simulink model "EKF_SIL_02"  (R2015a)
settings: Solver=ode45  StartTime=0.0  StopTime=totalSimulationTime  RelTol=1e-3
model workspace: external: MATLAB File Init_Model_02_Simulink.m (data not in the file)
undefined symbols (not defined in the file): Cov_nu, Cov_r, e_force_x, e_force_y, e_force_z, ieps, ita, lenLinks, n, P_d, P_k, p_x, p_y, p_z, parameter_gravitation, rho, rho_c, sig_f, sig_tau, t_delta, t_Kalman, tau_1, tau_2, tau_3, U_n_d, W_0, X_a_0, x_d, x_k
libraries: simulink x9, aerolibtransform2 x3, dspmtrx3 x2, visionstatistics x1, aerolibutil x1, visionsinks x1
(part 5 of 5)

== matlab function EKF_SIL_02/EKF/Measurement Update/Create X from X_a/Create del_q [Intermediate stage]/MATLAB Function ==
  data: q input; CrossTensor output; flag input
%Inputs: q: quaternion vector
%        flag:0-cross;1-star
function CrossTensor  = fn_CrossTensor(q,flag)
    %#codegen
    CrossTensor = zeros(4,4);
    q_v = q(1:3);
    q_0 = q(4);    
    cross_q_v = fn_VectorToSkewSymmetricTensor(q_v);
    switch (flag)
        case 0
            CrossTensor = [-cross_q_v + q_0*eye(3,3), q_v;-q_v',q_0];
        case 1
            CrossTensor = [cross_q_v + q_0*eye(3,3), q_v;-q_v',q_0];
        otherwise
            
    end
end

== matlab function EKF_SIL_02/EKF/Predictor/Create State error covariance (P)/State Propagation/MATLAB Function ==
  data: X_a input; Phi output; n input; t_Kalman input; p input; M input
%Function: fn_Create_Phi()
%Inputs: X_a - 23-state vector,
%        n - angular velocity of spacecrafts,
%        t_delta - sampling time
%Outputs: [Phi] (State-propagation Matrix)
%Functionality: Generates the State Propagation matrix
%Author: Hrishik Mishra
function Phi  = fn_Create_Phi(X_a,n,t_Kalman,p,M)
    Phi_t = fn_Create_Phi_t(n,t_Kalman);
    Phi_r = fn_Create_Phi_r(X_a,p, t_Kalman);
    Phi = [Phi_r, zeros(6,6);zeros(6,6),Phi_t];

end
%Create state propagation matrix of the whole system

%Function: fn_Create_Phi_r()
%Inputs: X_a - 23-state vector,
%Outputs: [Phi_r] (State-propagation Matrix for Rotation component)
%Functionality: Generates the State Propagation matrix for Rotation
%component
%Author: Hrishik Mishra
function [Phi_r] = fn_Create_Phi_r(X_a,p,t_Kalman) 
    Phi_r = zeros(6,6);
    omega = X_a(5:7);
    M = fn_Create_M(p,omega);   
    
    A = [-fn_VectorToSkewSymmetricTensor(omega),0.5*eye(3,3);zeros(3,3),M];
    Phi_r = expm(A*t_Kalman);
%     phi_r11 = fn_Create_phi_r11(omega,t_delta);
%     phi_r12 = fn_Create_phi_r12(omega,M,t_delta);
%     phi_r22 = fn_Create_phi_r22(omega,t_delta,M);
%     phi_r13 = fn_Create_phi_r13(omega,t_delta,M,N);
%     phi_r23 = fn_Create_phi_r23(omega,t_delta,M,N);
%     Phi_r = [phi_r11, phi_r12, phi_r13;zeros(3,3),phi_r22,phi_r23;zeros(3,3),zeros(3,3),eye(3,3)];
%     

end
%Function: fn_Create_M()
%Inputs: p - Inertial ratios 
%        omega - angular velocity between Chaser Grasping frame and Chaser
%        CoM
%Outputs: M (Linearized model matrix for inertial parameters)
%Functionality: Generates M
%Author: Hrishik Mishra
function M = fn_Create_M(p,omega)
    %#Codegen
    
    M = [0, p(1)*omega(3), p(1)*omega(2); p(2)*omega(3), 0, p(2)*omega(1); p(3)*omega(2),p(3)*omega(1),0];
end
%Function: fn_Create_N()
%Inputs: omega - angular velocity between Chaser Grasping frame and Chaser
%        CoM
%Outputs: N (Linearized model matrix for inertial parameters)
%Functionality: Generates M
%Author: Hrishik Mishra
function N = fn_Create_N(omega)
%
    N = [omega(2)*omega(3), 0, 0; 0, omega(1)*omega(3), 0; 0, 0, omega(1)*omega(2)];
end

%%
%Function: fn_Create_Phi_t()
%Inputs: n - angular velocity of Chaser/Target (almost same)
%        t_delta - sampling time
%Outputs: Phi_t (State Transition Matrix for Translation component)
%Functionality: Generates Phi_t
%Author: Hrishik Mishra
function Phi_t = fn_Create_Phi_t(n,t_delta)
%
    Phi_t12 = [t_delta, n*t_delta^2,0;0, t_delta, 0;0,0,t_delta];
    Phi_t22 = eye(3,3) - 2*fn_VectorToSkewSymmetricTensor([0;0;n])*t_delta;
    
    Phi_t = [eye(3,3),Phi_t12;zeros(3,3),Phi_t22];
    
end

== matlab function EKF_SIL_02/EKF/Predictor/Create State error covariance (P)/Process noise covariance [rotational]/Process Noise covariance ==
  data: Phi input; Q_r output; unused1 input; t_delta input; tau input; unused input; p input
%Function: fn_Create_Q_r()
%Inputs: Phi - State Propagation Matrix for Rotational component
%        X - 23-state vector
%        t_delta - sampling time
%        tau - Torque disturbance
%        sig_p - Uncertainty in Inertial ratios (p)
%Outputs: Q_r (Rotation component Process noise)
%Functionality: Generates Q_r
%Author: Hrishik Mishra
function Q_r = fn_Create_Q_r(Phi,~, t_delta, tau,~,p)
    %#codegen
    J = fn_Create_J(p);
    Q_r11 = 0.25*fn_Create_Q_r11(Phi(1:3,4:6), J, t_delta, tau);
    Q_r12 = 0.5*fn_Create_Q_r12(Phi(1:3,4:6),Phi(4:6,4:6),J,t_delta,tau);
    Q_r22 = fn_Create_Q_r22(Phi(4:6,4:6),J,t_delta,tau);
    Q_r = [Q_r11, Q_r12;Q_r12' Q_r22];
    
end
%check if it is actually phi_r12 or phi_r11
function Q_r11 = fn_Create_Q_r11(phi_r12, J, t_delta, tau)
    Q_r11 = tau*phi_r12*J^2*phi_r12'*t_delta; 
end

function Q_r12 = fn_Create_Q_r12(phi_r12,phi_r22,J, t_delta, tau)
    Q_r12 = tau*phi_r12*J^2*phi_r22*t_delta;
end
function Q_r22 = fn_Create_Q_r22(phi_r22, J, t_delta, tau)
    Q_r22 = tau*phi_r22*J^2*phi_r22*t_delta;
end
%Function: fn_Create_J()
%Inputs: p: Inertial ratios
%Outputs: J (Inertial Ratio Matrix for omega_dot)
%Functionality: Generates J
%Author: Hrishik Mishra
function J = fn_Create_J(p)
    J = [1 0 0;0 (1-p(2))/(1+p(1)) 0;0 0 (1+p(3))/(1-p(1))];
end

== matlab function EKF_SIL_02/EKF/Predictor/Create State error covariance (P)/Process noise covariance [translational]/Process noise covariance [translational] ==
  data: t_Kalman input; Q_t_k output; n input; sigma_f input
%Function: fn_Create_Q_t_k()
%Inputs: t_delta: sampling time
%        sigma_f: variance of force perturbations
%Outputs: Q_t_k (Translational component Process noise)
%Functionality: Generates Q_t_k
%Author: Hrishik Mishra
function Q_t_k  = fn_Create_Q_t_k(t_Kalman, n,sigma_f)
    %#codegen

    Q_t11_k = [(t_Kalman^3)/3 + (2/5)*n^2*t_Kalman^5, (1/4)*(n - n^2)*t_Kalman^4, 0;(1/4)*(n - n^2)*t_Kalman^4, (t_Kalman^3)/3 - (4/15)*n^2*t_Kalman^5 0;0, 0, (t_Kalman^3)/3 - (1/15)*n^2*t_Kalman^5];
    Q_t12_k = [(t_Kalman^2)/2 + (1/3)*(n^2)*(t_Kalman^4), -(1/3)*n*(t_Kalman^3),0;(2/3)*(n - n^2)*t_Kalman^3, (1/2)*(t_Kalman^2) - (2/3)*(n^2)*(t_Kalman^4) 0;0 0 (1/2)*(t_Kalman^2) - (1/6)*(n^2)*(t_Kalman^4)];
    Q_t22_k = [t_Kalman + (n^2)*(t_Kalman^3), 0, 0;0, t_Kalman, 0;0, 0, t_Kalman - (1/3)*(n^2)*(t_Kalman^3)];

    Q_t_k = [Q_t11_k, Q_t12_k;Q_t12_k',Q_t22_k];

    Q_t_k = sigma_f*Q_t_k;
end

== matlab function EKF_SIL_02/EKF/Measurement Update/Update with K(k) and predict current state/Create observation/MATLAB Function ==
  data: q input; CrossTensor output; flag input
%Inputs: q: quaternion vector
%        flag:0-cross;1-star
function CrossTensor  = fn_CrossTensor(q,flag)
    %#codegen
    CrossTensor = zeros(4,4);
    q_v = q(1:3);
    q_0 = q(4);    
    cross_q_v = fn_VectorToSkewSymmetricTensor(q_v);
    switch (flag)
        case 0
            CrossTensor = [-cross_q_v + q_0*eye(3,3), q_v;-q_v',q_0];
        case 1
            CrossTensor = [cross_q_v + q_0*eye(3,3), q_v;-q_v',q_0];
        otherwise
            
    end
end

== matlab function EKF_SIL_02/EKF/Measurement Update/Update with K(k) and predict current state/Measurement noise covariance ==
  data: q_nominal input; S output; ita_nominal input; cov_r input; cov_nu input
%Function: fn_Create_S()
%Inputs: q_nominal: Quaternion between Chaser CoM and Target CoM
%        ita_nominal: Quaternion between Target CoM and Target grasping
%        frame
%        cov_r: position covariance due to camera
%        cov_nu: orientation covariance due to camera
%Outputs: S (Measurement noise covariance Matrix)
%Functionality: Generates S
%Author: Hrishik Mishra
function S   = fn_Create_S(q_nominal,ita_nominal,cov_r,cov_nu)
    %#codegen
    q_star = [-q_nominal(1:3);q_nominal(4)];
    ita_star = [-ita_nominal(1:3);ita_nominal(4)];
    Ita_Tensor = fn_CrossTensor(ita_star,0);
    Q_Tensor = fn_CrossTensor(q_star,1);
    T = [eye(3,3),zeros(3,1)]*Ita_Tensor*Q_Tensor;
    S = [cov_r,zeros(3,3);zeros(3,3), T*cov_nu*T'];
end

== matlab function EKF_SIL_02/EKF/Measurement Update/Update with K(k) and predict current state/Create observation/MATLAB Function2 ==
  data: q input; CrossTensor output; flag input
%Inputs: q: quaternion vector
%        flag:0-cross;1-star
function CrossTensor  = fn_CrossTensor(q,flag)
    %#codegen
    CrossTensor = zeros(4,4);
    q_v = q(1:3);
    q_0 = q(4);    
    cross_q_v = fn_VectorToSkewSymmetricTensor(q_v);
    switch (flag)
        case 0
            CrossTensor = [-cross_q_v + q_0*eye(3,3), q_v;-q_v',q_0];
        case 1
            CrossTensor = [cross_q_v + q_0*eye(3,3), q_v;-q_v',q_0];
        otherwise
            
    end
end

== matlab function EKF_SIL_02/EKF/Measurement Update/Update with K(k) and predict current state/Create h/Subsystem/MATLAB Function2 ==
  data: q input; CrossTensor output; flag input
%Inputs: q: quaternion vector
%        flag:0-cross;1-star
function CrossTensor  = fn_CrossTensor(q,flag)
    %#codegen
    CrossTensor = zeros(4,4);
    q_v = q(1:3);
    q_0 = q(4);    
    cross_q_v = fn_VectorToSkewSymmetricTensor(q_v);
    switch (flag)
        case 0
            CrossTensor = [-cross_q_v + q_0*eye(3,3), q_v;-q_v',q_0];
        case 1
            CrossTensor = [cross_q_v + q_0*eye(3,3), q_v;-q_v',q_0];
        otherwise
            
    end
end

== matlab function EKF_SIL_02/EKF/Measurement Update/Update with K(k) and predict current state/Create X_a from X/Create q_nominal /MATLAB Function2 ==
  data: q input; CrossTensor output; flag input
%Inputs: q: quaternion vector
%        flag:0-cross;1-star
function CrossTensor  = fn_CrossTensor(q,flag)
    %#codegen
    CrossTensor = zeros(4,4);
    q_v = q(1:3);
    q_0 = q(4);    
    cross_q_v = fn_VectorToSkewSymmetricTensor(q_v);
    switch (flag)
        case 0
            CrossTensor = [-cross_q_v + q_0*eye(3,3), q_v;-q_v',q_0];
        case 1
            CrossTensor = [cross_q_v + q_0*eye(3,3), q_v;-q_v',q_0];
        otherwise
            
    end
end

== matlab function EKF_SIL_02/EKF/OOSM_KF/OOSM_KF/Initialize OOSM/Create State error covariance (P)/Process noise covariance [rotational]/Process Noise covariance ==
  data: Phi input; Q_r output; unused1 input; t_delta input; tau input; unused input; p input
%Function: fn_Create_Q_r()
%Inputs: Phi - State Propagation Matrix for Rotational component
%        X - 23-state vector
%        t_delta - sampling time
%        tau - Torque disturbance
%        sig_p - Uncertainty in Inertial ratios (p)
%Outputs: Q_r (Rotation component Process noise)
%Functionality: Generates Q_r
%Author: Hrishik Mishra
function Q_r = fn_Create_Q_r(Phi,~, t_delta, tau,~,p)
    %#codegen
    J = fn_Create_J(p);
    Q_r11 = 0.25*fn_Create_Q_r11(Phi(1:3,4:6), J, t_delta, tau);
    Q_r12 = 0.5*fn_Create_Q_r12(Phi(1:3,4:6),Phi(4:6,4:6),J,t_delta,tau);
    Q_r22 = fn_Create_Q_r22(Phi(4:6,4:6),J,t_delta,tau);
    Q_r = [Q_r11, Q_r12;Q_r12' Q_r22];
    
end
%check if it is actually phi_r12 or phi_r11
function Q_r11 = fn_Create_Q_r11(phi_r12, J, t_delta, tau)
    Q_r11 = tau*phi_r12*J^2*phi_r12'*t_delta; 
end

function Q_r12 = fn_Create_Q_r12(phi_r12,phi_r22,J, t_delta, tau)
    Q_r12 = tau*phi_r12*J^2*phi_r22*t_delta;
end
function Q_r22 = fn_Create_Q_r22(phi_r22, J, t_delta, tau)
    Q_r22 = tau*phi_r22*J^2*phi_r22*t_delta;
end
%Function: fn_Create_J()
%Inputs: p: Inertial ratios
%Outputs: J (Inertial Ratio Matrix for omega_dot)
%Functionality: Generates J
%Author: Hrishik Mishra
function J = fn_Create_J(p)
    J = [1 0 0;0 (1-p(2))/(1+p(1)) 0;0 0 (1+p(3))/(1-p(1))];
end

== matlab function EKF_SIL_02/Plots and display/Create Measurements [Pose]1/Create Measurements [Orientation] /MATLAB Function ==
  data: q input; CrossTensor output; flag input
%Inputs: q: quaternion vector
%        flag:0-cross;1-star
function CrossTensor  = fn_CrossTensor(q,flag)
    %#codegen
    CrossTensor = zeros(4,4);
    q_v = q(1:3);
    q_0 = q(4);    
    cross_q_v = fn_VectorToSkewSymmetricTensor(q_v);
    switch (flag)
        case 0
            CrossTensor = [-cross_q_v + q_0*eye(3,3), q_v;-q_v',q_0];
        case 1
            CrossTensor = [cross_q_v + q_0*eye(3,3), q_v;-q_v',q_0];
        otherwise
            
    end
end

== matlab function EKF_SIL_02/EKF/OOSM_KF/OOSM_KF/Initialize OOSM/Create State error covariance (P)/Process noise covariance [translational]/Process noise covariance [translational] ==
  data: t_Kalman input; Q_t_k output; n input; sigma_f input
%Function: fn_Create_Q_t_k()
%Inputs: t_delta: sampling time
%        sigma_f: variance of force perturbations
%Outputs: Q_t_k (Translational component Process noise)
%Functionality: Generates Q_t_k
%Author: Hrishik Mishra
function Q_t_k  = fn_Create_Q_t_k(t_Kalman, n,sigma_f)
    %#codegen

    Q_t11_k = [(t_Kalman^3)/3 + (2/5)*n^2*t_Kalman^5, (1/4)*(n - n^2)*t_Kalman^4, 0;(1/4)*(n - n^2)*t_Kalman^4, (t_Kalman^3)/3 - (4/15)*n^2*t_Kalman^5 0;0, 0, (t_Kalman^3)/3 - (1/15)*n^2*t_Kalman^5];
    Q_t12_k = [(t_Kalman^2)/2 + (1/3)*(n^2)*(t_Kalman^4), -(1/3)*n*(t_Kalman^3),0;(2/3)*(n - n^2)*t_Kalman^3, (1/2)*(t_Kalman^2) - (2/3)*(n^2)*(t_Kalman^4) 0;0 0 (1/2)*(t_Kalman^2) - (1/6)*(n^2)*(t_Kalman^4)];
    Q_t22_k = [t_Kalman + (n^2)*(t_Kalman^3), 0, 0;0, t_Kalman, 0;0, 0, t_Kalman - (1/3)*(n^2)*(t_Kalman^3)];

    Q_t_k = [Q_t11_k, Q_t12_k;Q_t12_k',Q_t22_k];

    Q_t_k = sigma_f*Q_t_k;
end

== matlab function EKF_SIL_02/EKF/OOSM_KF/OOSM_KF/Initialize OOSM/Create State error covariance (P)/State Propagation/MATLAB Function ==
  data: X_a input; Phi output; n input; t_Kalman input; p input; M input
%Function: fn_Create_Phi()
%Inputs: X_a - 23-state vector,
%        n - angular velocity of spacecrafts,
%        t_delta - sampling time
%Outputs: [Phi] (State-propagation Matrix)
%Functionality: Generates the State Propagation matrix
%Author: Hrishik Mishra
function Phi  = fn_Create_Phi(X_a,n,t_Kalman,p,M)
    Phi_t = fn_Create_Phi_t(n,t_Kalman);
    Phi_r = fn_Create_Phi_r(X_a,p, t_Kalman);
    Phi = [Phi_r, zeros(6,6);zeros(6,6),Phi_t];

end
%Create state propagation matrix of the whole system

%Function: fn_Create_Phi_r()
%Inputs: X_a - 23-state vector,
%Outputs: [Phi_r] (State-propagation Matrix for Rotation component)
%Functionality: Generates the State Propagation matrix for Rotation
%component
%Author: Hrishik Mishra
function [Phi_r] = fn_Create_Phi_r(X_a,p,t_Kalman) 
    Phi_r = zeros(6,6);
    omega = X_a(4:6);
    M = fn_Create_M(p,omega);   
    
    A = [-fn_VectorToSkewSymmetricTensor(omega),0.5*eye(3,3);zeros(3,3),M];
    Phi_r = expm(A*t_Kalman);
%     phi_r11 = fn_Create_phi_r11(omega,t_delta);
%     phi_r12 = fn_Create_phi_r12(omega,M,t_delta);
%     phi_r22 = fn_Create_phi_r22(omega,t_delta,M);
%     phi_r13 = fn_Create_phi_r13(omega,t_delta,M,N);
%     phi_r23 = fn_Create_phi_r23(omega,t_delta,M,N);
%     Phi_r = [phi_r11, phi_r12, phi_r13;zeros(3,3),phi_r22,phi_r23;zeros(3,3),zeros(3,3),eye(3,3)];
%     

end
%Function: fn_Create_M()
%Inputs: p - Inertial ratios 
%        omega - angular velocity between Chaser Grasping frame and Chaser
%        CoM
%Outputs: M (Linearized model matrix for inertial parameters)
%Functionality: Generates M
%Author: Hrishik Mishra
function M = fn_Create_M(p,omega)
    %#Codegen
    
    M = [0, p(1)*omega(3), p(1)*omega(2); p(2)*omega(3), 0, p(2)*omega(1); p(3)*omega(2),p(3)*omega(1),0];
end
%Function: fn_Create_N()
%Inputs: omega - angular velocity between Chaser Grasping frame and Chaser
%        CoM
%Outputs: N (Linearized model matrix for inertial parameters)
%Functionality: Generates M
%Author: Hrishik Mishra
function N = fn_Create_N(omega)
%
    N = [omega(2)*omega(3), 0, 0; 0, omega(1)*omega(3), 0; 0, 0, omega(1)*omega(2)];
end

%%
%Function: fn_Create_Phi_t()
%Inputs: n - angular velocity of Chaser/Target (almost same)
%        t_delta - sampling time
%Outputs: Phi_t (State Transition Matrix for Translation component)
%Functionality: Generates Phi_t
%Author: Hrishik Mishra
function Phi_t = fn_Create_Phi_t(n,t_delta)
%
    Phi_t12 = [t_delta, n*t_delta^2,0;0, t_delta, 0;0,0,t_delta];
    Phi_t22 = eye(3,3) - 2*fn_VectorToSkewSymmetricTensor([0;0;n])*t_delta;
    
    Phi_t = [eye(3,3),Phi_t12;zeros(3,3),Phi_t22];
    
end

== matlab function EKF_SIL_02/EKF/Predictor/Dynamic Model (Differential equations)2/Dynamic Model (Differential equations)/Quaternion Kinematics/MATLAB Function ==
  data: q input; CrossTensor output; flag input
%Inputs: q: quaternion vector
%        flag:0-cross;1-star
function CrossTensor  = fn_CrossTensor(q,flag)
    %#codegen
    CrossTensor = zeros(4,4);
    q_v = q(1:3);
    q_0 = q(4);    
    cross_q_v = fn_VectorToSkewSymmetricTensor(q_v);
    switch (flag)
        case 0
            CrossTensor = [-cross_q_v + q_0*eye(3,3), q_v;-q_v',q_0];
        case 1
            CrossTensor = [cross_q_v + q_0*eye(3,3), q_v;-q_v',q_0];
        otherwise
            
    end
end

== matlab function EKF_SIL_02/Plots and display/Create Measurements [Pose]2/Create Measurements [Orientation] /MATLAB Function ==
  data: q input; CrossTensor output; flag input
%Inputs: q: quaternion vector
%        flag:0-cross;1-star
function CrossTensor  = fn_CrossTensor(q,flag)
    %#codegen
    CrossTensor = zeros(4,4);
    q_v = q(1:3);
    q_0 = q(4);    
    cross_q_v = fn_VectorToSkewSymmetricTensor(q_v);
    switch (flag)
        case 0
            CrossTensor = [-cross_q_v + q_0*eye(3,3), q_v;-q_v',q_0];
        case 1
            CrossTensor = [cross_q_v + q_0*eye(3,3), q_v;-q_v',q_0];
        otherwise
            
    end
end

== matlab function EKF_SIL_02/EKF/Measurement Update/Update with K(k) and predict current state/Create observation/MATLAB Function1 ==
  data: q input; CrossTensor output; flag input
%Inputs: q: quaternion vector
%        flag:0-cross;1-star
function CrossTensor  = fn_CrossTensor(q,flag)
    %#codegen
    CrossTensor = zeros(4,4);
    q_v = q(1:3);
    q_0 = q(4);    
    cross_q_v = fn_VectorToSkewSymmetricTensor(q_v);
    switch (flag)
        case 0
            CrossTensor = [-cross_q_v + q_0*eye(3,3), q_v;-q_v',q_0];
        case 1
            CrossTensor = [cross_q_v + q_0*eye(3,3), q_v;-q_v',q_0];
        otherwise
            
    end
end

== matlab function EKF_SIL_02/EKF/OOSM_KF/OOSM_KF/Initialize OOSM/Propagate_state (full)/State Propagation1/MATLAB Function ==
  data: X_a input; Phi output; n input; t_Kalman input; p input; M input
%Function: fn_Create_Phi()
%Inputs: X_a - 23-state vector,
%        n - angular velocity of spacecrafts,
%        t_delta - sampling time
%Outputs: [Phi] (State-propagation Matrix)
%Functionality: Generates the State Propagation matrix
%Author: Hrishik Mishra
function Phi  = fn_Create_Phi(X_a,n,t_Kalman,p,M)
    Phi_t = fn_Create_Phi_t(n,t_Kalman);
    Phi_r = fn_Create_Phi_r(X_a,p, t_Kalman);
    Phi = [Phi_r, zeros(6,6);zeros(6,6),Phi_t];

end
%Create state propagation matrix of the whole system

%Function: fn_Create_Phi_r()
%Inputs: X_a - 23-state vector,
%Outputs: [Phi_r] (State-propagation Matrix for Rotation component)
%Functionality: Generates the State Propagation matrix for Rotation
%component
%Author: Hrishik Mishra
function [Phi_r] = fn_Create_Phi_r(X_a,p,t_Kalman) 
    Phi_r = zeros(6,6);
    omega = X_a(4:6);
    M = fn_Create_M(p,omega);   
    
    A = [-fn_VectorToSkewSymmetricTensor(omega),0.5*eye(3,3);zeros(3,3),M];
    Phi_r = expm(A*t_Kalman);
%     phi_r11 = fn_Create_phi_r11(omega,t_delta);
%     phi_r12 = fn_Create_phi_r12(omega,M,t_delta);
%     phi_r22 = fn_Create_phi_r22(omega,t_delta,M);
%     phi_r13 = fn_Create_phi_r13(omega,t_delta,M,N);
%     phi_r23 = fn_Create_phi_r23(omega,t_delta,M,N);
%     Phi_r = [phi_r11, phi_r12, phi_r13;zeros(3,3),phi_r22,phi_r23;zeros(3,3),zeros(3,3),eye(3,3)];
%     

end
%Function: fn_Create_M()
%Inputs: p - Inertial ratios 
%        omega - angular velocity between Chaser Grasping frame and Chaser
%        CoM
%Outputs: M (Linearized model matrix for inertial parameters)
%Functionality: Generates M
%Author: Hrishik Mishra
function M = fn_Create_M(p,omega)
    %#Codegen
    
    M = [0, p(1)*omega(3), p(1)*omega(2); p(2)*omega(3), 0, p(2)*omega(1); p(3)*omega(2),p(3)*omega(1),0];
end
%Function: fn_Create_N()
%Inputs: omega - angular velocity between Chaser Grasping frame and Chaser
%        CoM
%Outputs: N (Linearized model matrix for inertial parameters)
%Functionality: Generates M
%Author: Hrishik Mishra
function N = fn_Create_N(omega)
%
    N = [omega(2)*omega(3), 0, 0; 0, omega(1)*omega(3), 0; 0, 0, omega(1)*omega(2)];
end

%%
%Function: fn_Create_Phi_t()
%Inputs: n - angular velocity of Chaser/Target (almost same)
%        t_delta - sampling time
%Outputs: Phi_t (State Transition Matrix for Translation component)
%Functionality: Generates Phi_t
%Author: Hrishik Mishra
function Phi_t = fn_Create_Phi_t(n,t_delta)
%
    Phi_t12 = [t_delta, n*t_delta^2,0;0, t_delta, 0;0,0,t_delta];
    Phi_t22 = eye(3,3) - 2*fn_VectorToSkewSymmetricTensor([0;0;n])*t_delta;
    
    Phi_t = [eye(3,3),Phi_t12;zeros(3,3),Phi_t22];
    
end

== matlab function EKF_SIL_02/EKF/OOSM_KF/OOSM_KF/Initialize OOSM/State Propagation/MATLAB Function ==
  data: X_a input; Phi output; n input; t_Kalman input; p input; M input
%Function: fn_Create_Phi()
%Inputs: X_a - 23-state vector,
%        n - angular velocity of spacecrafts,
%        t_delta - sampling time
%Outputs: [Phi] (State-propagation Matrix)
%Functionality: Generates the State Propagation matrix
%Author: Hrishik Mishra
function Phi  = fn_Create_Phi(X_a,n,t_Kalman,p,M)
    Phi_t = fn_Create_Phi_t(n,t_Kalman);
    Phi_r = fn_Create_Phi_r(X_a,p, t_Kalman);
    Phi = [Phi_r, zeros(6,6);zeros(6,6),Phi_t];

end
%Create state propagation matrix of the whole system

%Function: fn_Create_Phi_r()
%Inputs: X_a - 23-state vector,
%Outputs: [Phi_r] (State-propagation Matrix for Rotation component)
%Functionality: Generates the State Propagation matrix for Rotation
%component
%Author: Hrishik Mishra
function [Phi_r] = fn_Create_Phi_r(X_a,p,t_Kalman) 
    Phi_r = zeros(6,6);
    omega = X_a(4:6);
    M = fn_Create_M(p,omega);   
    
    A = [-fn_VectorToSkewSymmetricTensor(omega),0.5*eye(3,3);zeros(3,3),M];
    Phi_r = expm(A*t_Kalman);
%     phi_r11 = fn_Create_phi_r11(omega,t_delta);
%     phi_r12 = fn_Create_phi_r12(omega,M,t_delta);
%     phi_r22 = fn_Create_phi_r22(omega,t_delta,M);
%     phi_r13 = fn_Create_phi_r13(omega,t_delta,M,N);
%     phi_r23 = fn_Create_phi_r23(omega,t_delta,M,N);
%     Phi_r = [phi_r11, phi_r12, phi_r13;zeros(3,3),phi_r22,phi_r23;zeros(3,3),zeros(3,3),eye(3,3)];
%     

end
%Function: fn_Create_M()
%Inputs: p - Inertial ratios 
%        omega - angular velocity between Chaser Grasping frame and Chaser
%        CoM
%Outputs: M (Linearized model matrix for inertial parameters)
%Functionality: Generates M
%Author: Hrishik Mishra
function M = fn_Create_M(p,omega)
    %#Codegen
    
    M = [0, p(1)*omega(3), p(1)*omega(2); p(2)*omega(3), 0, p(2)*omega(1); p(3)*omega(2),p(3)*omega(1),0];
end
%Function: fn_Create_N()
%Inputs: omega - angular velocity between Chaser Grasping frame and Chaser
%        CoM
%Outputs: N (Linearized model matrix for inertial parameters)
%Functionality: Generates M
%Author: Hrishik Mishra
function N = fn_Create_N(omega)
%
    N = [omega(2)*omega(3), 0, 0; 0, omega(1)*omega(3), 0; 0, 0, omega(1)*omega(2)];
end

%%
%Function: fn_Create_Phi_t()
%Inputs: n - angular velocity of Chaser/Target (almost same)
%        t_delta - sampling time
%Outputs: Phi_t (State Transition Matrix for Translation component)
%Functionality: Generates Phi_t
%Author: Hrishik Mishra
function Phi_t = fn_Create_Phi_t(n,t_delta)
%
    Phi_t12 = [t_delta, n*t_delta^2,0;0, t_delta, 0;0,0,t_delta];
    Phi_t22 = eye(3,3) - 2*fn_VectorToSkewSymmetricTensor([0;0;n])*t_delta;
    
    Phi_t = [eye(3,3),Phi_t12;zeros(3,3),Phi_t22];
    
end

== matlab function EKF_SIL_02/EKF/OOSM_KF/OOSM_KF/State Propagation1/MATLAB Function ==
  data: X_a input; Phi output; n input; t_Kalman input; p input; M input
%Function: fn_Create_Phi()
%Inputs: X_a - 23-state vector,
%        n - angular velocity of spacecrafts,
%        t_delta - sampling time
%Outputs: [Phi] (State-propagation Matrix)
%Functionality: Generates the State Propagation matrix
%Author: Hrishik Mishra
function Phi  = fn_Create_Phi(X_a,n,t_Kalman,p,M)
    Phi_t = fn_Create_Phi_t(n,t_Kalman);
    Phi_r = fn_Create_Phi_r(X_a,p, t_Kalman);
    Phi = [Phi_r, zeros(6,6);zeros(6,6),Phi_t];

end
%Create state propagation matrix of the whole system

%Function: fn_Create_Phi_r()
%Inputs: X_a - 23-state vector,
%Outputs: [Phi_r] (State-propagation Matrix for Rotation component)
%Functionality: Generates the State Propagation matrix for Rotation
%component
%Author: Hrishik Mishra
function [Phi_r] = fn_Create_Phi_r(X_a,p,t_Kalman) 
    Phi_r = zeros(6,6);
    omega = X_a(5:7);
    M = fn_Create_M(p,omega);   
    
    A = [-fn_VectorToSkewSymmetricTensor(omega),0.5*eye(3,3);zeros(3,3),M];
    Phi_r = expm(A*t_Kalman);
%     phi_r11 = fn_Create_phi_r11(omega,t_delta);
%     phi_r12 = fn_Create_phi_r12(omega,M,t_delta);
%     phi_r22 = fn_Create_phi_r22(omega,t_delta,M);
%     phi_r13 = fn_Create_phi_r13(omega,t_delta,M,N);
%     phi_r23 = fn_Create_phi_r23(omega,t_delta,M,N);
%     Phi_r = [phi_r11, phi_r12, phi_r13;zeros(3,3),phi_r22,phi_r23;zeros(3,3),zeros(3,3),eye(3,3)];
%     

end
%Function: fn_Create_M()
%Inputs: p - Inertial ratios 
%        omega - angular velocity between Chaser Grasping frame and Chaser
%        CoM
%Outputs: M (Linearized model matrix for inertial parameters)
%Functionality: Generates M
%Author: Hrishik Mishra
function M = fn_Create_M(p,omega)
    %#Codegen
    
    M = [0, p(1)*omega(3), p(1)*omega(2); p(2)*omega(3), 0, p(2)*omega(1); p(3)*omega(2),p(3)*omega(1),0];
end
%Function: fn_Create_N()
%Inputs: omega - angular velocity between Chaser Grasping frame and Chaser
%        CoM
%Outputs: N (Linearized model matrix for inertial parameters)
%Functionality: Generates M
%Author: Hrishik Mishra
function N = fn_Create_N(omega)
%
    N = [omega(2)*omega(3), 0, 0; 0, omega(1)*omega(3), 0; 0, 0, omega(1)*omega(2)];
end

%%
%Function: fn_Create_Phi_t()
%Inputs: n - angular velocity of Chaser/Target (almost same)
%        t_delta - sampling time
%Outputs: Phi_t (State Transition Matrix for Translation component)
%Functionality: Generates Phi_t
%Author: Hrishik Mishra
function Phi_t = fn_Create_Phi_t(n,t_delta)
%
    Phi_t12 = [t_delta, n*t_delta^2,0;0, t_delta, 0;0,0,t_delta];
    Phi_t22 = eye(3,3) - 2*fn_VectorToSkewSymmetricTensor([0;0;n])*t_delta;
    
    Phi_t = [eye(3,3),Phi_t12;zeros(3,3),Phi_t22];
    
end

== matlab function EKF_SIL_02/EKF/Measurement Update/Update with K(d) and update current state/Measurement noise covariance (t_d) ==
  data: q_nominal input; S output; ita_nominal input; cov_r input; cov_nu input
%Function: fn_Create_S()
%Inputs: q_nominal: Quaternion between Chaser CoM and Target CoM
%        ita_nominal: Quaternion between Target CoM and Target grasping
%        frame
%        cov_r: position covariance due to camera
%        cov_nu: orientation covariance due to camera
%Outputs: S (Measurement noise covariance Matrix)
%Functionality: Generates S
%Author: Hrishik Mishra
function S   = fn_Create_S(q_nominal,ita_nominal,cov_r,cov_nu)
    %#codegen
    q_star = [-q_nominal(1:3);q_nominal(4)];
    ita_star = [-ita_nominal(1:3);ita_nominal(4)];
    Ita_Tensor = fn_CrossTensor(ita_star,0);
    Q_Tensor = fn_CrossTensor(q_star,1);
    T = [eye(3,3),zeros(3,1)]*Ita_Tensor*Q_Tensor;
    S = [cov_r,zeros(3,3);zeros(3,3), T*cov_nu*T'];
end

== matlab function EKF_SIL_02/EKF/Measurement Update/Update with K(d) and update current state/Create observation1/MATLAB Function ==
  data: q input; CrossTensor output; flag input
%Inputs: q: quaternion vector
%        flag:0-cross;1-star
function CrossTensor  = fn_CrossTensor(q,flag)
    %#codegen
    CrossTensor = zeros(4,4);
    q_v = q(1:3);
    q_0 = q(4);    
    cross_q_v = fn_VectorToSkewSymmetricTensor(q_v);
    switch (flag)
        case 0
            CrossTensor = [-cross_q_v + q_0*eye(3,3), q_v;-q_v',q_0];
        case 1
            CrossTensor = [cross_q_v + q_0*eye(3,3), q_v;-q_v',q_0];
        otherwise
            
    end
end

== matlab function EKF_SIL_02/EKF/Measurement Update/Update with K(k) and predict current state/Propagate_state (full)/Create q_nominal/Create nominal q/MATLAB Function ==
  data: q input; CrossTensor output; flag input
%Inputs: q: quaternion vector
%        flag:0-cross;1-star
function CrossTensor  = fn_CrossTensor(q,flag)
    %#codegen
    CrossTensor = zeros(4,4);
    q_v = q(1:3);
    q_0 = q(4);    
    cross_q_v = fn_VectorToSkewSymmetricTensor(q_v);
    switch (flag)
        case 0
            CrossTensor = [-cross_q_v + q_0*eye(3,3), q_v;-q_v',q_0];
        case 1
            CrossTensor = [cross_q_v + q_0*eye(3,3), q_v;-q_v',q_0];
        otherwise
            
    end
end

== matlab function EKF_SIL_02/EKF/Measurement Update/Update with K(k) and predict current state/Propagate_state (full)/Create q_nominal/Create nominal q/MATLAB Function1 ==
  data: A input; exponent_A output
function exponent_A = fcn(A)
%#codegen
    exponent_A = expm(A);
end

== matlab function EKF_SIL_02/EKF/Predictor/Dynamic Model (Differential equations)1/Dynamic Model (Differential equations)/Quaternion Kinematics/MATLAB Function ==
  data: q input; CrossTensor output; flag input
%Inputs: q: quaternion vector
%        flag:0-cross;1-star
function CrossTensor  = fn_CrossTensor(q,flag)
    %#codegen
    CrossTensor = zeros(4,4);
    q_v = q(1:3);
    q_0 = q(4);    
    cross_q_v = fn_VectorToSkewSymmetricTensor(q_v);
    switch (flag)
        case 0
            CrossTensor = [-cross_q_v + q_0*eye(3,3), q_v;-q_v',q_0];
        case 1
            CrossTensor = [cross_q_v + q_0*eye(3,3), q_v;-q_v',q_0];
        otherwise
            
    end
end

== matlab function EKF_SIL_02/EKF/Measurement Update/Update with K(d) and update current state/Create observation1/MATLAB Function2 ==
  data: q input; CrossTensor output; flag input
%Inputs: q: quaternion vector
%        flag:0-cross;1-star
function CrossTensor  = fn_CrossTensor(q,flag)
    %#codegen
    CrossTensor = zeros(4,4);
    q_v = q(1:3);
    q_0 = q(4);    
    cross_q_v = fn_VectorToSkewSymmetricTensor(q_v);
    switch (flag)
        case 0
            CrossTensor = [-cross_q_v + q_0*eye(3,3), q_v;-q_v',q_0];
        case 1
            CrossTensor = [cross_q_v + q_0*eye(3,3), q_v;-q_v',q_0];
        otherwise
            
    end
end

== matlab function EKF_SIL_02/EKF/Measurement Update/Update with K(d) and update current state/Create h_d/Subsystem/MATLAB Function2 ==
  data: q input; CrossTensor output; flag input
%Inputs: q: quaternion vector
%        flag:0-cross;1-star
function CrossTensor  = fn_CrossTensor(q,flag)
    %#codegen
    CrossTensor = zeros(4,4);
    q_v = q(1:3);
    q_0 = q(4);    
    cross_q_v = fn_VectorToSkewSymmetricTensor(q_v);
    switch (flag)
        case 0
            CrossTensor = [-cross_q_v + q_0*eye(3,3), q_v;-q_v',q_0];
        case 1
            CrossTensor = [cross_q_v + q_0*eye(3,3), q_v;-q_v',q_0];
        otherwise
            
    end
end

== matlab function EKF_SIL_02/EKF/Predictor/Dynamic Model (Differential equations)2/Dynamic Model (Differential equations)/Pose Servicer base//EE/MATLAB Function ==
  data: len input; J output; ang input
function J = J(len,ang)
%J
%    OUT1 = J(IN1,IN2)

%    This function was generated by the Symbolic Math Toolbox version 6.0.
%    21-Jan-2017 11:55:10

l_3 = len(3,:);
l_4 = len(4,:);
l_5 = len(5,:);
l_6 = len(6,:);
l_7 = len(7,:);
q_1 = ang(1,:);
q_2 = ang(2,:);
q_3 = ang(3,:);
q_4 = ang(4,:);
q_5 = ang(5,:);
q_6 = ang(6,:);
t2 = pi.*q_1.*(1.0./1.8e2);
t3 = sin(t2);
t4 = pi.*q_3.*(1.0./1.8e2);
t5 = q_2+9.0e1;
t6 = pi.*t5.*(1.0./1.8e2);
t7 = q_4+9.0e1;
t8 = pi.*t7.*(1.0./1.8e2);
t9 = cos(t4);
t10 = sin(t6);
t11 = sin(t4);
t12 = cos(t6);
t13 = q_5+1.8e2;
t14 = pi.*t13.*(1.0./1.8e2);
t15 = cos(t8);
t16 = pi.*t3.*t9.*t10.*(1.0./1.8e2);
t17 = pi.*t3.*t11.*t12.*(1.0./1.8e2);
t18 = t16+t17;
t19 = sin(t8);
t20 = pi.*t3.*t9.*t12.*(1.0./1.8e2);
t44 = pi.*t3.*t10.*t11.*(1.0./1.8e2);
t21 = t20-t44;
t22 = cos(t2);
t23 = sin(t14);
t24 = pi.*t9.*t12.*t22.*(1.0./1.8e2);
t29 = pi.*t10.*t11.*t22.*(1.0./1.8e2);
t25 = t24-t29;
t26 = pi.*t9.*t10.*t22.*(1.0./1.8e2);
t27 = pi.*t11.*t12.*t22.*(1.0./1.8e2);
t28 = t26+t27;
t30 = t15.*t25;
t42 = t19.*t28;
t43 = t30-t42;
t31 = l_6.*t43;
t32 = t19.*t25;
t33 = t15.*t28;
t34 = t32+t33;
t35 = t9.*t10.*t22;
t36 = t11.*t12.*t22;
t37 = t35+t36;
t38 = t9.*t12.*t22;
t41 = t10.*t11.*t22;
t39 = t38-t41;
t40 = cos(t14);
t45 = t15.*t21;
t50 = t18.*t19;
t46 = t45-t50;
t47 = t15.*t18;
t48 = t19.*t21;
t49 = t47+t48;
t51 = l_6.*t46;
t52 = t3.*t9.*t10;
t53 = t3.*t11.*t12;
t54 = t52+t53;
t55 = t3.*t9.*t12;
t57 = t3.*t10.*t11;
t56 = t55-t57;
t58 = pi.*t9.*t10.*(1.0./1.8e2);
t59 = pi.*t11.*t12.*(1.0./1.8e2);
t60 = t58+t59;
t61 = pi.*t9.*t12.*(1.0./1.8e2);
t63 = pi.*t10.*t11.*(1.0./1.8e2);
t62 = t61-t63;
t64 = t19.*t62;
t65 = t15.*t60;
t66 = t64+t65;
t67 = l_6.*t66;
t68 = t15.*t62;
t102 = t19.*t60;
t140 = t68-t102;
t69 = l_7.*t23.*t140;
t70 = pi.*l_4.*t9.*t12.*(1.0./1.8e2);
t71 = t9.*t12;
t76 = t10.*t11;
t72 = t71-t76;
t73 = t9.*t10;
t74 = t11.*t12;
t75 = t73+t74;
t77 = pi.*q_6.*(1.0./1.8e2);
t78 = sin(t77);
t79 = cos(t77);
t80 = t78.*(t30-t42);
t81 = t80-t34.*t40.*t79;
t82 = pi.*t15.*t39.*(1.0./1.8e2);
t119 = pi.*t19.*t37.*(1.0./1.8e2);
t83 = t82-t119;
t84 = pi.*t15.*t37.*(1.0./1.8e2);
t85 = pi.*t19.*t39.*(1.0./1.8e2);
t86 = t84+t85;
t87 = t15.*t39;
t89 = t19.*t37;
t88 = t87-t89;
t90 = pi.*t3.*t23.*(1.0./1.8e2);
t91 = t46.*t78;
t92 = t91-t40.*t49.*t79;
t93 = pi.*t15.*t56.*(1.0./1.8e2);
t133 = pi.*t19.*t54.*(1.0./1.8e2);
t94 = t93-t133;
t95 = pi.*t15.*t54.*(1.0./1.8e2);
t96 = pi.*t19.*t56.*(1.0./1.8e2);
t97 = t95+t96;
t98 = t15.*t56;
t101 = t19.*t54;
t99 = t98-t101;
t100 = pi.*t22.*t40.*(1.0./1.8e2);
t103 = t66.*t78;
t104 = t40.*t79.*(t68-t102);
t105 = t103+t104;
t106 = pi.*t15.*t75.*(1.0./1.8e2);
t107 = pi.*t19.*t72.*(1.0./1.8e2);
t108 = t106+t107;
t109 = pi.*t15.*t72.*(1.0./1.8e2);
t143 = pi.*t19.*t75.*(1.0./1.8e2);
t110 = t109-t143;
t111 = t15.*t75;
t112 = t19.*t72;
t113 = t111+t112;
t114 = t40.*t46;
t115 = pi.*t22.*t23.*(1.0./1.8e2);
t116 = t79.*(t30-t42);
t117 = t34.*t40.*t78;
t118 = t116+t117;
t120 = pi.*t3.*t40.*(1.0./1.8e2);
t121 = t120-pi.*t23.*t88.*(1.0./1.8e2);
t122 = t15.*t37;
t123 = t19.*t39;
t124 = t122+t123;
t125 = t40.*t88;
t126 = t3.*t23;
t127 = t125+t126;
t128 = t40.*t43;
t129 = t90+t128;
t130 = t46.*t79;
t131 = t40.*t49.*t78;
t132 = t130+t131;
t134 = pi.*t23.*t99.*(1.0./1.8e2);
t135 = t100+t134;
t136 = t22.*t23;
t137 = t15.*t54;
t138 = t19.*t56;
t139 = t137+t138;
t141 = t66.*t79;
t142 = t141-t40.*t78.*t140;
t144 = t15.*t72;
t145 = t144-t19.*t75;
t146 = t23.*t46;
t147 = pi.*t40.*t88.*(1.0./1.8e2);
t148 = t90+t147;
t149 = t23.*(t68-t102);
J = reshape([-l_7.*(t100+t146)-l_6.*t49+pi.*l_5.*t22.*(1.0./1.8e2)-pi.*l_3.*t3.*t12.*(1.0./1.8e2)-pi.*l_4.*t3.*t9.*t12.*(1.0./1.8e2)+pi.*l_4.*t3.*t10.*t11.*(1.0./1.8e2),l_7.*(t23.*t43-pi.*t3.*t40.*(1.0./1.8e2))+l_6.*t34+pi.*l_5.*t3.*(1.0./1.8e2)+pi.*l_3.*t12.*t22.*(1.0./1.8e2)+pi.*l_4.*t9.*t12.*t22.*(1.0./1.8e2)-pi.*l_4.*t10.*t11.*t22.*(1.0./1.8e2),0.0,-t79.*(t114-pi.*t22.*t23.*(1.0./1.8e2))-t49.*t78,t34.*t78+t79.*t129,0.0,-t49.*t79+t78.*(t114-t115),t34.*t79-t78.*t129,0.0,-t100-t146,-t120+t23.*(t30-t42),0.0,t31-l_7.*t23.*t34-pi.*l_3.*t10.*t22.*(1.0./1.8e2)-pi.*l_4.*t9.*t10.*t22.*(1.0./1.8e2)-pi.*l_4.*t11.*t12.*t22.*(1.0./1.8e2),t51-l_7.*t23.*t49-pi.*l_3.*t3.*t10.*(1.0./1.8e2)-pi.*l_4.*t3.*t9.*t10.*(1.0./1.8e2)-pi.*l_4.*t3.*t11.*t12.*(1.0./1.8e2),t67+t69+t70+pi.*l_3.*t12.*(1.0./1.8e2)-pi.*l_4.*t10.*t11.*(1.0./1.8e2),t81,t92,t105,t118,t132,t142,-t23.*t34,-t23.*t49,t149,t31-l_7.*t23.*t34-pi.*l_4.*t9.*t10.*t22.*(1.0./1.8e2)-pi.*l_4.*t11.*t12.*t22.*(1.0./1.8e2),t51-l_7.*t23.*t49-pi.*l_4.*t3.*t9.*t10.*(1.0./1.8e2)-pi.*l_4.*t3.*t11.*t12.*(1.0./1.8e2),t67+t69+t70-pi.*l_4.*t10.*t11.*(1.0./1.8e2),t81,t92,t105,t118,t132,t142,-t23.*t34,-t23.*t49,t149,l_6.*t83-l_7.*t23.*t86,l_6.*t94-l_7.*t23.*t97,l_6.*t108+l_7.*t23.*t110,t78.*t83-t40.*t79.*t86,t78.*t94-t40.*t79.*t97,t78.*t108+t40.*t79.*t110,t79.*t83+t40.*t78.*t86,t79.*t94+t40.*t78.*t97,t79.*t108-t40.*t78.*t110,-t23.*t86,-t23.*t97,t23.*t110,l_7.*t148,-l_7.*(t115-pi.*t40.*t99.*(1.0./1.8e2)),pi.*l_7.*t40.*t113.*(1.0./1.8e2),t79.*t121,-t79.*t135,pi.*t23.*t79.*t113.*(-1.0./1.8e2),-t78.*t121,t78.*t135,pi.*t23.*t78.*t113.*(1.0./1.8e2),t148,-t115+pi.*t40.*t99.*(1.0./1.8e2),pi.*t40.*t113.*(1.0./1.8e2),0.0,0.0,0.0,pi.*t79.*t124.*(1.0./1.8e2)-pi.*t78.*t127.*(1.0./1.8e2),pi.*t78.*(t136-t40.*t99).*(1.0./1.8e2)+pi.*t79.*t139.*(1.0./1.8e2),pi.*t79.*t145.*(-1.0./1.8e2)-pi.*t40.*t78.*t113.*(1.0./1.8e2),pi.*t78.*t124.*(-1.0./1.8e2)-pi.*t79.*t127.*(1.0./1.8e2),pi.*t79.*(t136-t40.*t99).*(1.0./1.8e2)-pi.*t78.*t139.*(1.0./1.8e2),pi.*t78.*t145.*(1.0./1.8e2)-pi.*t40.*t79.*t113.*(1.0./1.8e2),0.0,0.0,0.0],[12, 6]);

== matlab function EKF_SIL_02/EKF/Measurement Update/Update with K(k) and predict current state/Propagate_state (full)/State Propagation1/MATLAB Function ==
  data: X_a input; Phi output; n input; t_Kalman input; p input; M input
%Function: fn_Create_Phi()
%Inputs: X_a - 23-state vector,
%        n - angular velocity of spacecrafts,
%        t_delta - sampling time
%Outputs: [Phi] (State-propagation Matrix)
%Functionality: Generates the State Propagation matrix
%Author: Hrishik Mishra
function Phi  = fn_Create_Phi(X_a,n,t_Kalman,p,M)
    Phi_t = fn_Create_Phi_t(n,t_Kalman);
    Phi_r = fn_Create_Phi_r(X_a,p, t_Kalman);
    Phi = [Phi_r, zeros(6,6);zeros(6,6),Phi_t];

end
%Create state propagation matrix of the whole system

%Function: fn_Create_Phi_r()
%Inputs: X_a - 23-state vector,
%Outputs: [Phi_r] (State-propagation Matrix for Rotation component)
%Functionality: Generates the State Propagation matrix for Rotation
%component
%Author: Hrishik Mishra
function [Phi_r] = fn_Create_Phi_r(X_a,p,t_Kalman) 
    Phi_r = zeros(6,6);
    omega = X_a(5:7);
    M = fn_Create_M(p,omega);   
    
    A = [-fn_VectorToSkewSymmetricTensor(omega),0.5*eye(3,3);zeros(3,3),M];
    Phi_r = expm(A*t_Kalman);
%     phi_r11 = fn_Create_phi_r11(omega,t_delta);
%     phi_r12 = fn_Create_phi_r12(omega,M,t_delta);
%     phi_r22 = fn_Create_phi_r22(omega,t_delta,M);
%     phi_r13 = fn_Create_phi_r13(omega,t_delta,M,N);
%     phi_r23 = fn_Create_phi_r23(omega,t_delta,M,N);
%     Phi_r = [phi_r11, phi_r12, phi_r13;zeros(3,3),phi_r22,phi_r23;zeros(3,3),zeros(3,3),eye(3,3)];
%     

end
%Function: fn_Create_M()
%Inputs: p - Inertial ratios 
%        omega - angular velocity between Chaser Grasping frame and Chaser
%        CoM
%Outputs: M (Linearized model matrix for inertial parameters)
%Functionality: Generates M
%Author: Hrishik Mishra
function M = fn_Create_M(p,omega)
    %#Codegen
    
    M = [0, p(1)*omega(3), p(1)*omega(2); p(2)*omega(3), 0, p(2)*omega(1); p(3)*omega(2),p(3)*omega(1),0];
end
%Function: fn_Create_N()
%Inputs: omega - angular velocity between Chaser Grasping frame and Chaser
%        CoM
%Outputs: N (Linearized model matrix for inertial parameters)
%Functionality: Generates M
%Author: Hrishik Mishra
function N = fn_Create_N(omega)
%
    N = [omega(2)*omega(3), 0, 0; 0, omega(1)*omega(3), 0; 0, 0, omega(1)*omega(2)];
end

%%
%Function: fn_Create_Phi_t()
%Inputs: n - angular velocity of Chaser/Target (almost same)
%        t_delta - sampling time
%Outputs: Phi_t (State Transition Matrix for Translation component)
%Functionality: Generates Phi_t
%Author: Hrishik Mishra
function Phi_t = fn_Create_Phi_t(n,t_delta)
%
    Phi_t12 = [t_delta, n*t_delta^2,0;0, t_delta, 0;0,0,t_delta];
    Phi_t22 = eye(3,3) - 2*fn_VectorToSkewSymmetricTensor([0;0;n])*t_delta;
    
    Phi_t = [eye(3,3),Phi_t12;zeros(3,3),Phi_t22];
    
end

== matlab function EKF_SIL_02/EKF/Measurement Update/Update with K(d) and update current state/Create X_a from X1/Create q_nominal /MATLAB Function2 ==
  data: q input; CrossTensor output; flag input
%Inputs: q: quaternion vector
%        flag:0-cross;1-star
function CrossTensor  = fn_CrossTensor(q,flag)
    %#codegen
    CrossTensor = zeros(4,4);
    q_v = q(1:3);
    q_0 = q(4);    
    cross_q_v = fn_VectorToSkewSymmetricTensor(q_v);
    switch (flag)
        case 0
            CrossTensor = [-cross_q_v + q_0*eye(3,3), q_v;-q_v',q_0];
        case 1
            CrossTensor = [cross_q_v + q_0*eye(3,3), q_v;-q_v',q_0];
        otherwise
            
    end
end

== matlab function EKF_SIL_02/EKF/OOSM_KF/OOSM_enable/Create nominal q(d)/MATLAB Function ==
  data: q input; CrossTensor output; flag input
%Inputs: q: quaternion vector
%        flag:0-cross;1-star
function CrossTensor  = fn_CrossTensor(q,flag)
    %#codegen
    CrossTensor = zeros(4,4);
    q_v = q(1:3);
    q_0 = q(4);    
    cross_q_v = fn_VectorToSkewSymmetricTensor(q_v);
    switch (flag)
        case 0
            CrossTensor = [-cross_q_v + q_0*eye(3,3), q_v;-q_v',q_0];
        case 1
            CrossTensor = [cross_q_v + q_0*eye(3,3), q_v;-q_v',q_0];
        otherwise
            
    end
end

== matlab function EKF_SIL_02/EKF/OOSM_KF/OOSM_KF/Create X from X_a/Create del_q [Intermediate stage]/MATLAB Function ==
  data: q input; CrossTensor output; flag input
%Inputs: q: quaternion vector
%        flag:0-cross;1-star
function CrossTensor  = fn_CrossTensor(q,flag)
    %#codegen
    CrossTensor = zeros(4,4);
    q_v = q(1:3);
    q_0 = q(4);    
    cross_q_v = fn_VectorToSkewSymmetricTensor(q_v);
    switch (flag)
        case 0
            CrossTensor = [-cross_q_v + q_0*eye(3,3), q_v;-q_v',q_0];
        case 1
            CrossTensor = [cross_q_v + q_0*eye(3,3), q_v;-q_v',q_0];
        otherwise
            
    end
end

== matlab function EKF_SIL_02/EKF/MATLAB Function ==
  data: len input; T_ee output; theta input
function T_ee = T_ee(len,theta)
%T_EE
%    OUT1 = T_EE(IN1,IN2)

%    This function was generated by the Symbolic Math Toolbox version 6.0.
%    20-Feb-2017 20:48:05

l_1 = len(1,:);
l_2 = len(2,:);
l_3 = len(3,:);
l_4 = len(4,:);
l_5 = len(5,:);
l_6 = len(6,:);
l_7 = len(7,:);
q_1 = theta(1,:);
q_2 = theta(2,:);
q_3 = theta(3,:);
q_4 = theta(4,:);
q_5 = theta(5,:);
q_6 = theta(6,:);
t2 = pi.*q_1.*(1.0./1.8e2);
t3 = cos(t2);
t4 = pi.*q_3.*(1.0./1.8e2);
t5 = q_2+9.0e1;
t6 = pi.*t5.*(1.0./1.8e2);
t7 = q_4+9.0e1;
t8 = pi.*t7.*(1.0./1.8e2);
t9 = cos(t4);
t10 = cos(t6);
t11 = sin(t4);
t12 = sin(t6);
t13 = pi.*q_6.*(1.0./1.8e2);
t14 = cos(t8);
t15 = t3.*t9.*t10;
t25 = t3.*t11.*t12;
t16 = t15-t25;
t17 = sin(t8);
t18 = t3.*t9.*t12;
t19 = t3.*t10.*t11;
t20 = t18+t19;
t21 = q_5+1.8e2;
t22 = pi.*t21.*(1.0./1.8e2);
t23 = cos(t13);
t24 = t14.*t20;
t26 = t16.*t17;
t27 = t24+t26;
t28 = sin(t13);
t29 = cos(t22);
t30 = t14.*t16;
t37 = t17.*t20;
t31 = t30-t37;
t32 = t29.*t31;
t33 = sin(t2);
t34 = sin(t22);
t35 = t33.*t34;
t36 = t32+t35;
t38 = t31.*t34;
t39 = t38-t29.*t33;
t40 = t9.*t10.*t33;
t46 = t11.*t12.*t33;
t41 = t40-t46;
t42 = t9.*t12.*t33;
t43 = t10.*t11.*t33;
t44 = t42+t43;
t45 = t14.*t44;
t47 = t17.*t41;
t48 = t45+t47;
t49 = t14.*t41;
t52 = t17.*t44;
t50 = t49-t52;
t51 = t3.*t34;
t53 = t34.*t50;
t54 = t3.*t29;
t55 = t53+t54;
t56 = t9.*t12;
t57 = t10.*t11;
t58 = t56+t57;
t59 = t9.*t10;
t61 = t11.*t12;
t60 = t59-t61;
t62 = t14.*t60;
t67 = t17.*t58;
t63 = t62-t67;
t64 = t14.*t58;
t65 = t17.*t60;
t66 = t64+t65;
T_ee = reshape([t27.*t28+t23.*t36,t28.*t48-t23.*(t51-t29.*t50),-t28.*t63+t23.*t29.*t66,0.0,t23.*t27-t28.*t36,t23.*t48+t28.*(t51-t29.*t50),-t23.*t63-t28.*t29.*t66,0.0,t39,t55,t34.*t66,0.0,l_6.*t27+l_5.*t33+l_7.*t39+l_3.*t3.*t10+l_4.*t3.*t9.*t10-l_4.*t3.*t11.*t12,-l_5.*t3+l_6.*t48+l_7.*t55+l_3.*t10.*t33+l_4.*t9.*t10.*t33-l_4.*t11.*t12.*t33,l_1+l_2+l_3.*t12-l_6.*t63+l_4.*t9.*t12+l_4.*t10.*t11+l_7.*t34.*t66,1.0],[4, 4]);

== matlab function EKF_SIL_02/EKF/Predictor/Dynamic Model (Differential equations)2/Dynamic Model (Differential equations)/Pose Servicer base//EE/MATLAB Function1 ==
  data: q input; CrossTensor output; flag input
%Inputs: q: quaternion vector
%        flag:0-cross;1-star
function CrossTensor  = fn_CrossTensor(q,flag)
    %#codegen
    CrossTensor = zeros(4,4);
    q_v = q(1:3);
    q_0 = q(4);    
    cross_q_v = fn_VectorToSkewSymmetricTensor(q_v);
    switch (flag)
        case 0
            CrossTensor = [-cross_q_v + q_0*eye(3,3), q_v;-q_v',q_0];
        case 1
            CrossTensor = [cross_q_v + q_0*eye(3,3), q_v;-q_v',q_0];
        otherwise
            
    end
end
